simulink model "InitialModel_backup"  (R2020a)
settings: Solver=VariableStepAuto  StartTime=0.0  StopTime=20  RelTol=0.001
values from neighbouring files (symbols this model uses):
  Ax = 0.1    [Simulink1.m]
  Ay = 0.1    [Simulink1.m]
  Az = 0.1    [Simulink1.m]
  g = 9.81    [Simulink1.m]
  Ixx = 0.00365    [Simulink1.m]
  Iyy = 0.00368    [Simulink1.m]
  Izz = 0.00703    [Simulink1.m]
  Jyy = 0.0064    [Simulink1.m]
  k_F = 6.11e-8    (= 6.11e-08)    [Simulink1.m]
  k_M = 1.5e-9    (= 1.5e-09)    [Simulink1.m]
  l = 0.17    [Simulink1.m]
  m = 0.5    [Simulink1.m]
settings Model: Creator=o_belzil  LastModifiedBy=o_belzil
settings SolverCC: MaxConsecutiveZCs=10  MaxConsecutiveMinStep=100  ZeroCrossAlgorithm=Adaptive
settings DebuggingCC: MaskedZcDiagnostic=none  IgnoredZcDiagnostic=none  UniqueDataStoreMsg=error

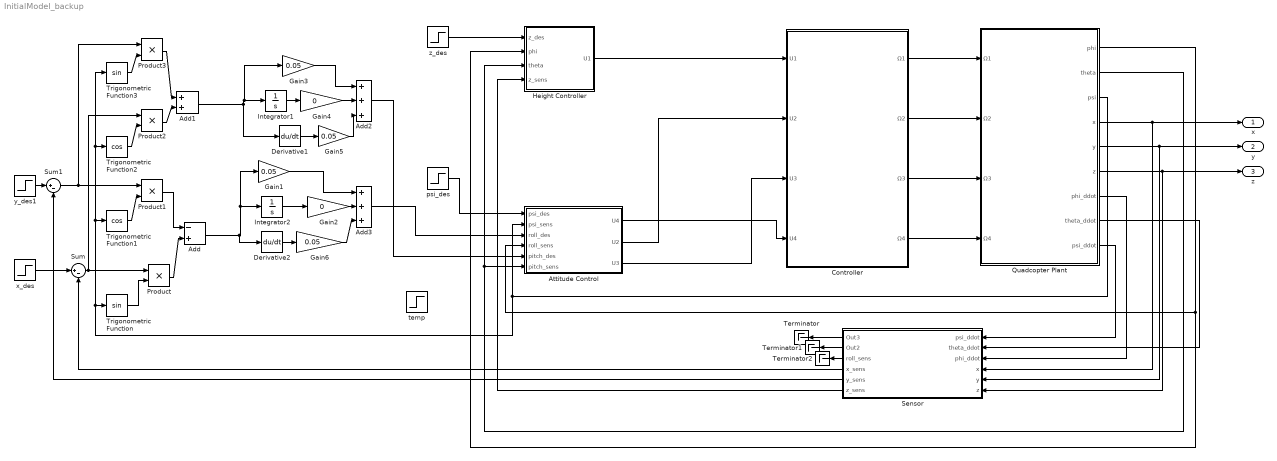
== system InitialModel_backup ==
  Add : Sum  Inputs=-+
  Add1 : Sum
  Add2 : Sum  Inputs=+++
  Add3 : Sum  Inputs=+++
  Attitude Control : Subsystem
  Controller : Subsystem
  Derivative1 : Derivative
  Derivative2 : Derivative
  Gain{1,3,5..6} (4 alike) : Gain  Gain=0.05
  Gain2 : Gain  Gain=0
  Gain4 : Gain  Gain=0
  Height Controller : Subsystem
  Integrator1 : Integrator
  Integrator2 : Integrator
  Product{,1..3} (4 alike) : Product
  Quadcopter Plant : Subsystem
  Sensor : Subsystem
  Sum : Sum  Inputs=|+-
  Sum1 : Sum  Inputs=|+-
  Terminator : Terminator
  Terminator1 : Terminator
  Terminator2 : Terminator
  Trigonometric Function : Trigonometry
  Trigonometric Function1 : Trigonometry  Operator=cos
  Trigonometric Function2 : Trigonometry  Operator=cos
  Trigonometric Function3 : Trigonometry
  psi_des : Step  Time=0  After=1.6  SampleTime=0
  temp : Step  Time=0  After=0.75  SampleTime=0
  x_des : Step  Time=2  After=5  SampleTime=0
  y_des1 : Step  Time=0  After=0  SampleTime=0
  z_des : Step  Time=0  After=10  SampleTime=0
  x : Outport
  y : Outport  Port=2
  z : Outport  Port=3
  wires:
  Quadcopter Plant/4(x) -> x/1, Sensor/4(x)
  Quadcopter Plant/5(y) -> y/1, Sensor/5(y)
  Quadcopter Plant/6(z) -> z/1, Sensor/6(z)
  Quadcopter Plant/7(phi_ddot) -> Sensor/3(phi_ddot)
  Quadcopter Plant/8(theta_ddot) -> Sensor/2(theta_ddot)
  Controller/1(Ω1) -> Quadcopter Plant/1(Ω1)
  Controller/2(Ω2) -> Quadcopter Plant/2(Ω2)
  Controller/3(Ω3) -> Quadcopter Plant/3(Ω3)
  Controller/4(Ω4) -> Quadcopter Plant/4(Ω4)
  Height Controller/1(U1) -> Controller/1(U1)
  z_des/1 -> Height Controller/1(z_des)
  Quadcopter Plant/1(phi) -> Attitude Control/4(roll_sens), Height Controller/2(phi)
  Quadcopter Plant/2(theta) -> Attitude Control/6(pitch_sens), Height Controller/3(theta)
  psi_des/1 -> Attitude Control/1(psi_des)
  Quadcopter Plant/3(psi) -> Attitude Control/2(psi_sens), Trigonometric Function3/1, Trigonometric Function2/1, Trigonometric Function1/1, Trigonometric Function/1
  Attitude Control/1(U4) -> Controller/4(U4)
  Sensor/6(z_sens) -> Height Controller/4(z_sens)
  Attitude Control/2(U2) -> Controller/2(U2)
  Attitude Control/3(U3) -> Controller/3(U3)
  x_des/1 -> Sum/1
  Sensor/4(x_sens) -> Sum/2
  Sum/1 -> Product/1, Product2/1
  Trigonometric Function/1 -> Product/2
  Product/1 -> Add/2
  y_des1/1 -> Sum1/1
  Sensor/5(y_sens) -> Sum1/2
  Sum1/1 -> Product1/1, Product3/1
  Trigonometric Function1/1 -> Product1/2
  Product1/1 -> Add/1
  Trigonometric Function2/1 -> Product2/2
  Trigonometric Function3/1 -> Product3/2
  Product3/1 -> Add1/1
  Product2/1 -> Add1/2
  Integrator1/1 -> Gain4/1
  Gain5/1 -> Add2/3
  Gain4/1 -> Add2/2
  Add1/1 -> Integrator1/1, Gain3/1, Derivative1/1
  Gain3/1 -> Add2/1
  Derivative1/1 -> Gain5/1
  Integrator2/1 -> Gain2/1
  Gain6/1 -> Add3/3
  Gain2/1 -> Add3/2
  Add/1 -> Derivative2/1, Integrator2/1, Gain1/1
  Gain1/1 -> Add3/1
  Derivative2/1 -> Gain6/1
  Sensor/2(Out2) -> Terminator1/1
  Sensor/3(roll_sens) -> Terminator2/1
  Sensor/1(Out3) -> Terminator/1
  Quadcopter Plant/9(psi_ddot) -> Sensor/1(psi_ddot)
  Add3/1 -> Attitude Control/3(roll_des)
  Add2/1 -> Attitude Control/5(pitch_des)

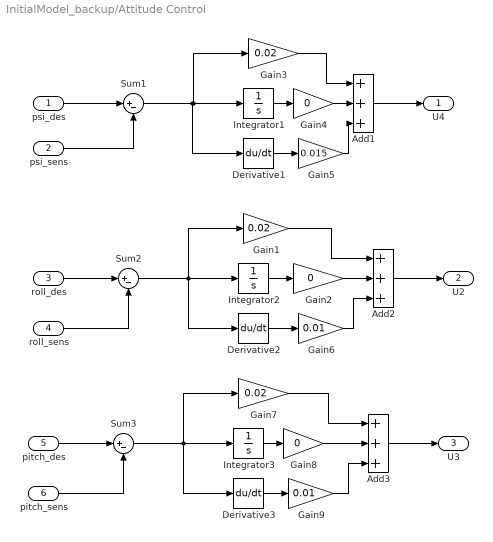
== system InitialModel_backup/Attitude Control ==
  psi_des : Inport
  psi_sens : Inport  Port=2
  roll_des : Inport  Port=3
  roll_sens : Inport  Port=4
  pitch_des : Inport  Port=5
  pitch_sens : Inport  Port=6
  Add1 : Sum  Inputs=+++
  Add2 : Sum  Inputs=+++
  Add3 : Sum  Inputs=+++
  Derivative1 : Derivative
  Derivative2 : Derivative
  Derivative3 : Derivative
  Gain1 : Gain  Gain=0.02
  Gain2 : Gain  Gain=0
  Gain3 : Gain  Gain=0.02
  Gain4 : Gain  Gain=0
  Gain5 : Gain  Gain=0.015
  Gain6 : Gain  Gain=0.01
  Gain7 : Gain  Gain=0.02
  Gain8 : Gain  Gain=0
  Gain9 : Gain  Gain=0.01
  Integrator1 : Integrator
  Integrator2 : Integrator
  Integrator3 : Integrator
  Sum1 : Sum  Inputs=|+-
  Sum2 : Sum  Inputs=|+-
  Sum3 : Sum  Inputs=|+-
  U4 : Outport
  U2 : Outport  Port=2
  U3 : Outport  Port=3
  wires:
  Gain3/1 -> Add1/1
  Gain4/1 -> Add1/2
  Gain5/1 -> Add1/3
  Derivative1/1 -> Gain5/1
  Integrator1/1 -> Gain4/1
  Add1/1 -> U4/1
  psi_des/1 -> Sum1/1
  psi_sens/1 -> Sum1/2
  Sum1/1 -> Derivative1/1, Integrator1/1, Gain3/1
  Integrator2/1 -> Gain2/1
  Gain6/1 -> Add2/3
  Gain2/1 -> Add2/2
  Add2/1 -> U2/1
  Sum2/1 -> Derivative2/1, Integrator2/1, Gain1/1
  roll_des/1 -> Sum2/1
  Gain1/1 -> Add2/1
  Derivative2/1 -> Gain6/1
  roll_sens/1 -> Sum2/2
  pitch_sens/1 -> Sum3/2
  Gain7/1 -> Add3/1
  Add3/1 -> U3/1
  Gain9/1 -> Add3/3
  Sum3/1 -> Derivative3/1, Integrator3/1, Gain7/1
  Integrator3/1 -> Gain8/1
  pitch_des/1 -> Sum3/1
  Gain8/1 -> Add3/2
  Derivative3/1 -> Gain9/1

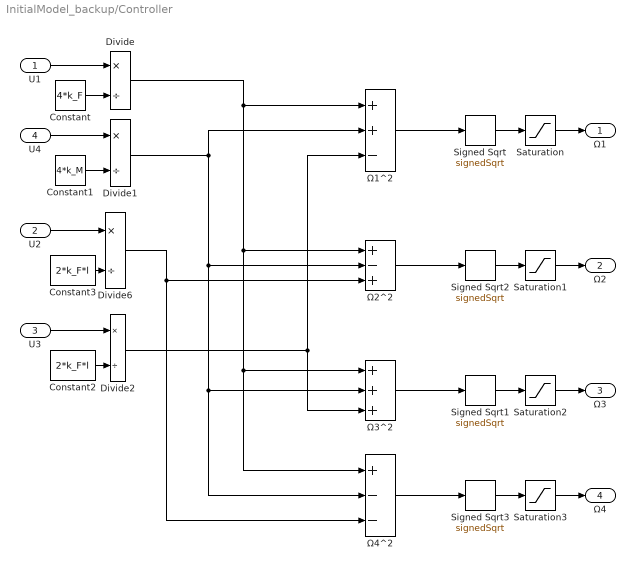
== system InitialModel_backup/Controller ==
  U1 : Inport
  U2 : Inport  Port=2
  U3 : Inport  Port=3
  U4 : Inport  Port=4
  Constant : Constant  Value=4*k_F
  Constant1 : Constant  Value=4*k_M
  Constant2 : Constant  Value=2*k_F*l
  Constant3 : Constant  Value=2*k_F*l
  Divide{,1..2,6} (4 alike) : Product  Inputs=*/
  Saturation{,1..3} (4 alike) : Saturate  UpperLimit=10000  LowerLimit=0
  Signed Sqrt{,1..3} (4 alike) : Sqrt  Operator=signedSqrt  SaturateOnIntegerOverflow=on
  Ω1^2 : Sum  Inputs=++-
  Ω2^2 : Sum  Inputs=+-+
  Ω3^2 : Sum  Inputs=+++
  Ω4^2 : Sum  Inputs=+--
  Ω1 : Outport
  Ω2 : Outport  Port=2
  Ω3 : Outport  Port=3
  Ω4 : Outport  Port=4
  wires:
  Ω1^2/1 -> Signed Sqrt/1
  Ω3^2/1 -> Signed Sqrt1/1
  Ω4^2/1 -> Signed Sqrt3/1
  Ω2^2/1 -> Signed Sqrt2/1
  U1/1 -> Divide/1
  Constant/1 -> Divide/2
  U4/1 -> Divide1/1
  Constant1/1 -> Divide1/2
  Constant2/1 -> Divide2/2
  U3/1 -> Divide2/1
  Constant3/1 -> Divide6/2
  U2/1 -> Divide6/1
  Divide/1 -> Ω4^2/1, Ω3^2/1, Ω2^2/1, Ω1^2/1
  Divide1/1 -> Ω4^2/2, Ω3^2/2, Ω2^2/2, Ω1^2/2
  Divide2/1 -> Ω3^2/3, Ω1^2/3
  Divide6/1 -> Ω4^2/3, Ω2^2/3
  Signed Sqrt3/1 -> Saturation3/1
  Saturation3/1 -> Ω4/1
  Signed Sqrt1/1 -> Saturation2/1
  Saturation2/1 -> Ω3/1
  Signed Sqrt2/1 -> Saturation1/1
  Saturation1/1 -> Ω2/1
  Signed Sqrt/1 -> Saturation/1
  Saturation/1 -> Ω1/1

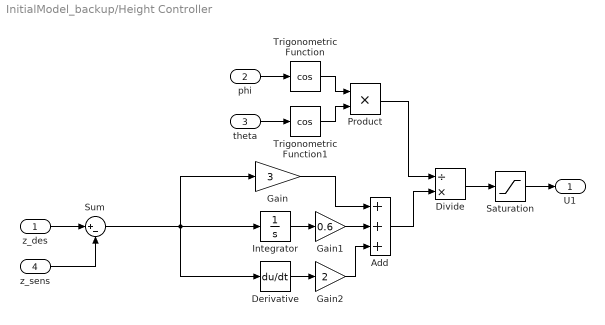
== system InitialModel_backup/Height Controller ==
  z_des : Inport
  phi : Inport  Port=2
  theta : Inport  Port=3
  z_sens : Inport  Port=4
  Add : Sum  Inputs=+++
  Derivative : Derivative
  Divide : Product  Inputs=/*
  Gain : Gain  Gain=3
  Gain1 : Gain  Gain=0.6
  Gain2 : Gain  Gain=2
  Integrator : Integrator
  Product : Product
  Saturation : Saturate  UpperLimit=inf  LowerLimit=0
  Sum : Sum  Inputs=|+-
  Trigonometric Function : Trigonometry  Operator=cos
  Trigonometric Function1 : Trigonometry  Operator=cos
  U1 : Outport
  wires:
  Integrator/1 -> Gain1/1
  Gain1/1 -> Add/2
  Trigonometric Function1/1 -> Product/2
  Derivative/1 -> Gain2/1
  Divide/1 -> Saturation/1
  Trigonometric Function/1 -> Product/1
  Gain/1 -> Add/1
  Product/1 -> Divide/1
  Gain2/1 -> Add/3
  Saturation/1 -> U1/1
  z_des/1 -> Sum/1
  z_sens/1 -> Sum/2
  phi/1 -> Trigonometric Function/1
  theta/1 -> Trigonometric Function1/1
  Sum/1 -> Integrator/1, Derivative/1, Gain/1
  Add/1 -> Divide/2

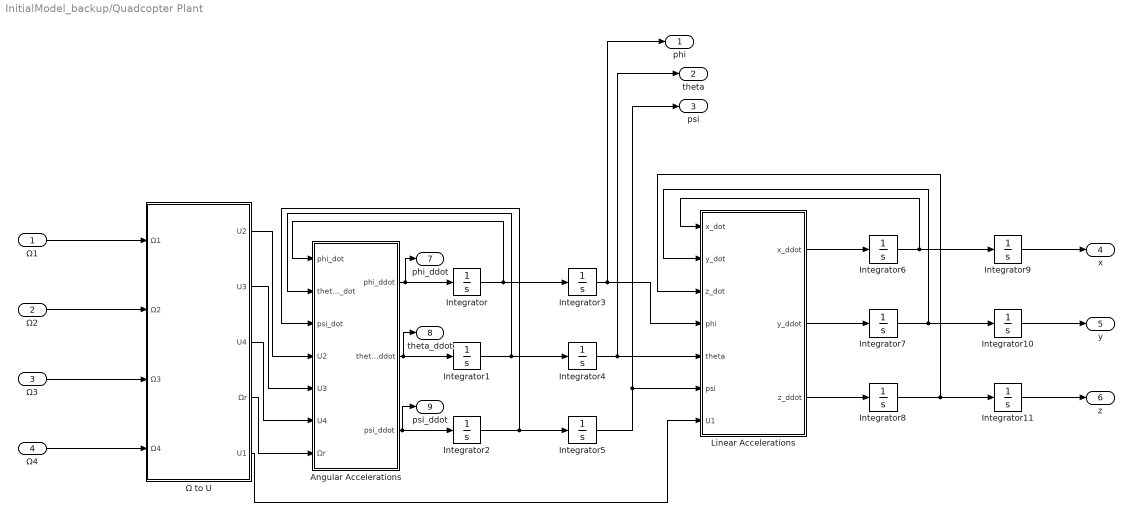
== system InitialModel_backup/Quadcopter Plant ==
  Ω1 : Inport
  Ω2 : Inport  Port=2
  Ω3 : Inport  Port=3
  Ω4 : Inport  Port=4
  Angular Accelerations : Subsystem
  Integrator{,1..2,6..10} (8 alike) : Integrator
  Integrator11 : Integrator  LimitOutput=on  LowerSaturationLimit=0
  Integrator3 : Integrator  WrapState=on
  Integrator4 : Integrator  WrapState=on
  Integrator5 : Integrator  WrapState=on
  Linear Accelerations : Subsystem
  Ω to U : Subsystem
  phi : Outport
  theta : Outport  Port=2
  psi : Outport  Port=3
  x : Outport  Port=4
  y : Outport  Port=5
  z : Outport  Port=6
  phi_ddot : Outport  Port=7
  theta_ddot : Outport  Port=8
  psi_ddot : Outport  Port=9
  wires:
  Ω1/1 -> Ω to U/1(Ω1)
  Ω2/1 -> Ω to U/2(Ω2)
  Ω3/1 -> Ω to U/3(Ω3)
  Ω4/1 -> Ω to U/4(Ω4)
  Ω to U/1(U2) -> Angular Accelerations/4(U2)
  Ω to U/2(U3) -> Angular Accelerations/5(U3)
  Ω to U/3(U4) -> Angular Accelerations/6(U4)
  Ω to U/4(Ωr) -> Angular Accelerations/7(Ωr)
  Angular Accelerations/3(psi_ddot) -> psi_ddot/1, Integrator2/1
  Angular Accelerations/2(theta_ddot) -> Integrator1/1, theta_ddot/1
  Angular Accelerations/1(phi_ddot) -> phi_ddot/1, Integrator/1
  Integrator/1 -> Integrator3/1, Angular Accelerations/1(phi_dot)
  Integrator1/1 -> Integrator4/1, Angular Accelerations/2(theta_dot)
  Integrator2/1 -> Integrator5/1, Angular Accelerations/3(psi_dot)
  Integrator3/1 -> Linear Accelerations/4(phi), phi/1
  Integrator4/1 -> Linear Accelerations/5(theta), theta/1
  Integrator5/1 -> psi/1, Linear Accelerations/6(psi)
  Linear Accelerations/1(x_ddot) -> Integrator6/1
  Linear Accelerations/2(y_ddot) -> Integrator7/1
  Linear Accelerations/3(z_ddot) -> Integrator8/1
  Integrator6/1 -> Integrator9/1, Linear Accelerations/1(x_dot)
  Integrator7/1 -> Integrator10/1, Linear Accelerations/2(y_dot)
  Integrator8/1 -> Integrator11/1, Linear Accelerations/3(z_dot)
  Integrator9/1 -> x/1
  Integrator10/1 -> y/1
  Integrator11/1 -> z/1
  Ω to U/5(U1) -> Linear Accelerations/7(U1)

== system InitialModel_backup/Sensor ==
  psi_ddot : Inport
  theta_ddot : Inport  Port=2
  phi_ddot : Inport  Port=3
  x : Inport  Port=4
  y : Inport  Port=5
  z : Inport  Port=6
  Out3 : Outport
  Out2 : Outport  Port=2
  roll_sens : Outport  Port=3
  x_sens : Outport  Port=4
  y_sens : Outport  Port=5
  z_sens : Outport  Port=6
  wires:
  phi_ddot/1 -> roll_sens/1
  theta_ddot/1 -> Out2/1
  psi_ddot/1 -> Out3/1
  x/1 -> x_sens/1
  z/1 -> z_sens/1
  y/1 -> y_sens/1

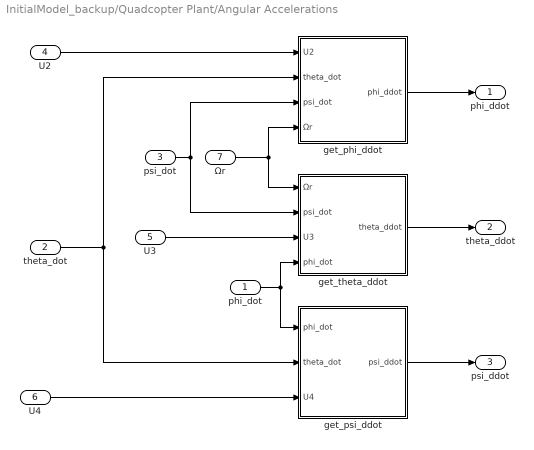
== system InitialModel_backup/Quadcopter Plant/Angular Accelerations ==
  phi_dot : Inport
  theta_dot : Inport  Port=2
  psi_dot : Inport  Port=3
  U2 : Inport  Port=4
  U3 : Inport  Port=5
  U4 : Inport  Port=6
  Ωr : Inport  Port=7
  get_phi_ddot : Subsystem
  get_psi_ddot : Subsystem
  get_theta_ddot : Subsystem
  phi_ddot : Outport
  theta_ddot : Outport  Port=2
  psi_ddot : Outport  Port=3
  wires:
  get_phi_ddot/1(phi_ddot) -> phi_ddot/1
  get_theta_ddot/1(theta_ddot) -> theta_ddot/1
  get_psi_ddot/1(psi_ddot) -> psi_ddot/1
  U2/1 -> get_phi_ddot/1(U2)
  U4/1 -> get_psi_ddot/3(U4)
  Ωr/1 -> get_theta_ddot/1(Ωr), get_phi_ddot/4(Ωr)
  psi_dot/1 -> get_theta_ddot/2(psi_dot), get_phi_ddot/3(psi_dot)
  phi_dot/1 -> get_psi_ddot/1(phi_dot), get_theta_ddot/4(phi_dot)
  theta_dot/1 -> get_psi_ddot/2(theta_dot), get_phi_ddot/2(theta_dot)
  U3/1 -> get_theta_ddot/3(U3)

== system InitialModel_backup/Quadcopter Plant/Linear Accelerations ==
  x_dot : Inport
  y_dot : Inport  Port=2
  z_dot : Inport  Port=3
  phi : Inport  Port=4
  theta : Inport  Port=5
  psi : Inport  Port=6
  U1 : Inport  Port=7
  get_x_ddot : Subsystem
  get_y_ddot : Subsystem
  get_z_ddot : Subsystem
  x_ddot : Outport
  y_ddot : Outport  Port=2
  z_ddot : Outport  Port=3
  wires:
  x_dot/1 -> get_x_ddot/1(x_dot)
  y_dot/1 -> get_y_ddot/1(y_dot)
  z_dot/1 -> get_z_ddot/1(z_dot)
  psi/1 -> get_x_ddot/4(psi), get_y_ddot/4(psi)
  theta/1 -> get_z_ddot/3(theta), get_y_ddot/3(theta), get_x_ddot/3(theta)
  phi/1 -> get_x_ddot/2(phi), get_z_ddot/2(phi), get_y_ddot/2(phi)
  get_z_ddot/1(z_ddot) -> z_ddot/1
  get_y_ddot/1(y_ddot) -> y_ddot/1
  get_x_ddot/1(x_ddot) -> x_ddot/1
  U1/1 -> get_z_ddot/4(U1), get_y_ddot/5(U1), get_x_ddot/5(U1)

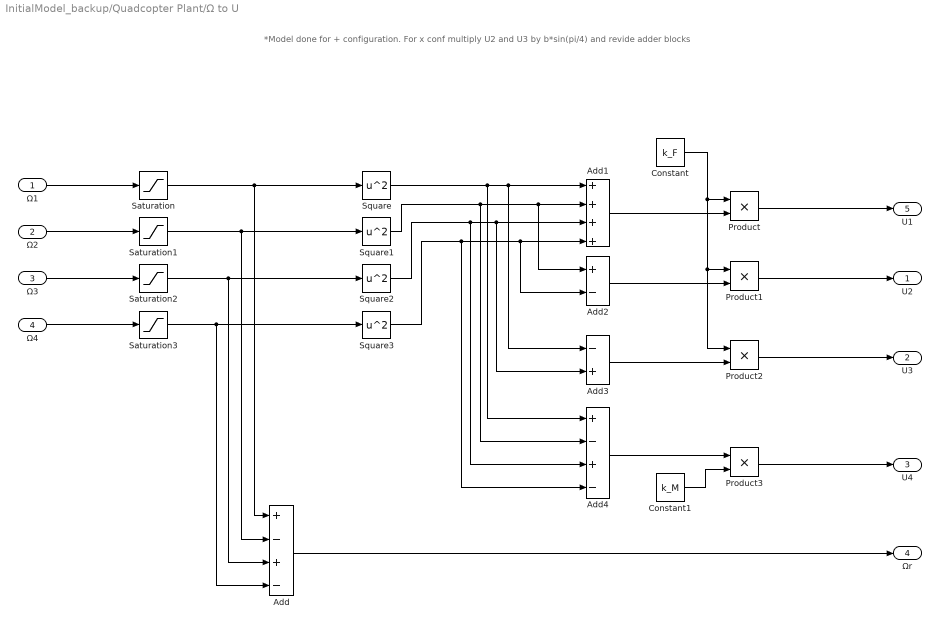
== system InitialModel_backup/Quadcopter Plant/Ω to U ==
  note: *Model done for + configuration. For x conf multiply U2 and U3 by b*sin(pi/4) and revide adder blocks
  Ω1 : Inport
  Ω2 : Inport  Port=2
  Ω3 : Inport  Port=3
  Ω4 : Inport  Port=4
  Add : Sum  Inputs=+-+-
  Add1 : Sum  Inputs=++++
  Add2 : Sum  Inputs=+-
  Add3 : Sum  Inputs=-+
  Add4 : Sum  Inputs=+-+-
  Constant : Constant  Value=k_F
  Constant1 : Constant  Value=k_M
  Product{,1..3} (4 alike) : Product
  Saturation{,1..3} (4 alike) : Saturate  UpperLimit=inf  LowerLimit=0
  Square{,1..3} (4 alike) : Math  Operator=square  SaturateOnIntegerOverflow=on
  U2 : Outport
  U3 : Outport  Port=2
  U4 : Outport  Port=3
  Ωr : Outport  Port=4
  U1 : Outport  Port=5
  wires:
  Ω1/1 -> Saturation/1
  Ω2/1 -> Saturation1/1
  Ω3/1 -> Saturation2/1
  Ω4/1 -> Saturation3/1
  Add/1 -> Ωr/1
  Square/1 -> Add3/1, Add1/1, Add4/1
  Square1/1 -> Add2/1, Add1/2, Add4/2
  Square2/1 -> Add3/2, Add1/3, Add4/3
  Square3/1 -> Add4/4, Add2/2, Add1/4
  Add1/1 -> Product/2
  Add2/1 -> Product1/2
  Add3/1 -> Product2/2
  Add4/1 -> Product3/1
  Constant1/1 -> Product3/2
  Constant/1 -> Product/1, Product2/1, Product1/1
  Product/1 -> U1/1
  Product1/1 -> U2/1
  Product2/1 -> U3/1
  Product3/1 -> U4/1
  Saturation/1 -> Square/1, Add/1
  Saturation1/1 -> Square1/1, Add/2
  Saturation2/1 -> Square2/1, Add/3
  Saturation3/1 -> Square3/1, Add/4

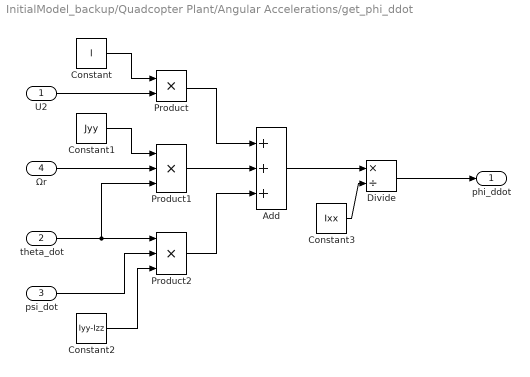
== system InitialModel_backup/Quadcopter Plant/Angular Accelerations/get_phi_ddot ==
  U2 : Inport
  theta_dot : Inport  Port=2
  psi_dot : Inport  Port=3
  Ωr : Inport  Port=4
  Add : Sum  Inputs=+++
  Constant : Constant  Value=l
  Constant1 : Constant  Value=Jyy
  Constant2 : Constant  Value=Iyy-Izz
  Constant3 : Constant  Value=Ixx
  Divide : Product  Inputs=*/
  Product : Product
  Product1 : Product  Inputs=3
  Product2 : Product  Inputs=3
  phi_ddot : Outport
  wires:
  U2/1 -> Product/2
  Constant/1 -> Product/1
  Ωr/1 -> Product1/2
  Constant1/1 -> Product1/1
  theta_dot/1 -> Product2/1, Product1/3
  psi_dot/1 -> Product2/2
  Constant2/1 -> Product2/3
  Product/1 -> Add/1
  Product1/1 -> Add/2
  Product2/1 -> Add/3
  Add/1 -> Divide/1
  Constant3/1 -> Divide/2
  Divide/1 -> phi_ddot/1

== system InitialModel_backup/Quadcopter Plant/Angular Accelerations/get_psi_ddot ==
  phi_dot : Inport
  theta_dot : Inport  Port=2
  U4 : Inport  Port=3
  Add : Sum
  Constant : Constant  Value=Ixx-Iyy
  Constant1 : Constant  Value=Izz
  Divide : Product  Inputs=*/
  Product : Product  Inputs=3
  psi_ddot : Outport
  wires:
  Constant1/1 -> Divide/2
  Add/1 -> Divide/1
  U4/1 -> Add/1
  phi_dot/1 -> Product/1
  theta_dot/1 -> Product/2
  Constant/1 -> Product/3
  Product/1 -> Add/2
  Divide/1 -> psi_ddot/1

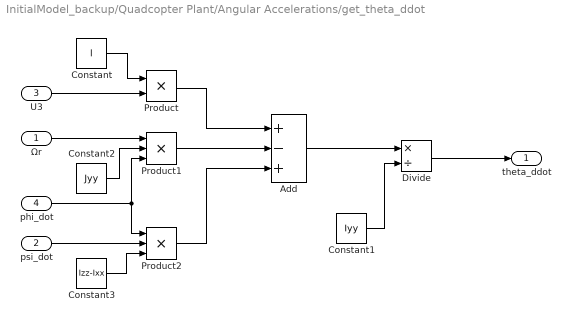
== system InitialModel_backup/Quadcopter Plant/Angular Accelerations/get_theta_ddot ==
  Ωr : Inport
  psi_dot : Inport  Port=2
  U3 : Inport  Port=3
  phi_dot : Inport  Port=4
  Add : Sum  Inputs=+-+
  Constant : Constant  Value=l
  Constant1 : Constant  Value=Iyy
  Constant2 : Constant  Value=Jyy
  Constant3 : Constant  Value=Izz-Ixx
  Divide : Product  Inputs=*/
  Product : Product
  Product1 : Product  Inputs=3
  Product2 : Product  Inputs=3
  theta_ddot : Outport
  wires:
  Constant/1 -> Product/1
  U3/1 -> Product/2
  Ωr/1 -> Product1/1
  phi_dot/1 -> Product2/1, Product1/3
  Constant2/1 -> Product1/2
  Constant3/1 -> Product2/3
  psi_dot/1 -> Product2/2
  Product/1 -> Add/1
  Product1/1 -> Add/2
  Product2/1 -> Add/3
  Add/1 -> Divide/1
  Constant1/1 -> Divide/2
  Divide/1 -> theta_ddot/1

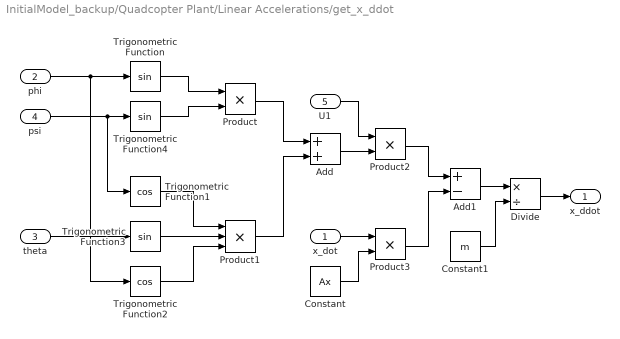
== system InitialModel_backup/Quadcopter Plant/Linear Accelerations/get_x_ddot ==
  x_dot : Inport
  phi : Inport  Port=2
  theta : Inport  Port=3
  psi : Inport  Port=4
  U1 : Inport  Port=5
  Add : Sum
  Add1 : Sum  Inputs=+-
  Constant : Constant  Value=Ax
  Constant1 : Constant  Value=m
  Divide : Product  Inputs=*/
  Product : Product
  Product1 : Product  Inputs=3
  Product2 : Product
  Product3 : Product
  Trigonometric Function : Trigonometry
  Trigonometric Function1 : Trigonometry  Operator=cos
  Trigonometric Function2 : Trigonometry  Operator=cos
  Trigonometric Function3 : Trigonometry
  Trigonometric Function4 : Trigonometry
  x_ddot : Outport
  wires:
  phi/1 -> Trigonometric Function2/1, Trigonometric Function/1
  psi/1 -> Trigonometric Function1/1, Trigonometric Function4/1
  theta/1 -> Trigonometric Function3/1
  Trigonometric Function/1 -> Product/1
  Trigonometric Function4/1 -> Product/2
  Trigonometric Function3/1 -> Product1/2
  Trigonometric Function1/1 -> Product1/1
  Trigonometric Function2/1 -> Product1/3
  Product/1 -> Add/1
  Product1/1 -> Add/2
  Add/1 -> Product2/2
  U1/1 -> Product2/1
  x_dot/1 -> Product3/1
  Constant/1 -> Product3/2
  Product2/1 -> Add1/1
  Product3/1 -> Add1/2
  Add1/1 -> Divide/1
  Constant1/1 -> Divide/2
  Divide/1 -> x_ddot/1

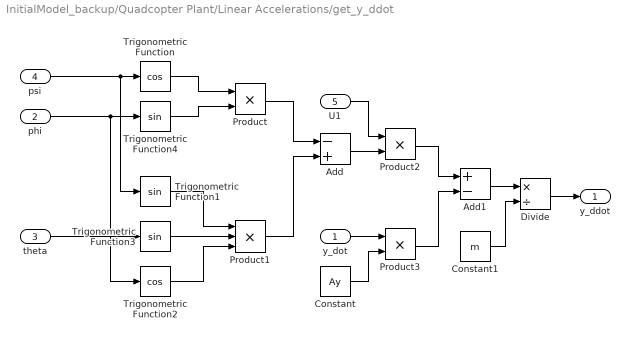
== system InitialModel_backup/Quadcopter Plant/Linear Accelerations/get_y_ddot ==
  y_dot : Inport
  phi : Inport  Port=2
  theta : Inport  Port=3
  psi : Inport  Port=4
  U1 : Inport  Port=5
  Add : Sum  Inputs=-+
  Add1 : Sum  Inputs=+-
  Constant : Constant  Value=Ay
  Constant1 : Constant  Value=m
  Divide : Product  Inputs=*/
  Product : Product
  Product1 : Product  Inputs=3
  Product2 : Product
  Product3 : Product
  Trigonometric Function : Trigonometry  Operator=cos
  Trigonometric Function1 : Trigonometry
  Trigonometric Function2 : Trigonometry  Operator=cos
  Trigonometric Function3 : Trigonometry
  Trigonometric Function4 : Trigonometry
  y_ddot : Outport
  wires:
  Trigonometric Function4/1 -> Product/2
  Trigonometric Function3/1 -> Product1/2
  Trigonometric Function1/1 -> Product1/1
  Add1/1 -> Divide/1
  Product1/1 -> Add/2
  Divide/1 -> y_ddot/1
  y_dot/1 -> Product3/1
  Trigonometric Function/1 -> Product/1
  Product/1 -> Add/1
  Constant/1 -> Product3/2
  Constant1/1 -> Divide/2
  Product2/1 -> Add1/1
  U1/1 -> Product2/1
  Product3/1 -> Add1/2
  Trigonometric Function2/1 -> Product1/3
  Add/1 -> Product2/2
  phi/1 -> Trigonometric Function2/1, Trigonometric Function4/1
  psi/1 -> Trigonometric Function1/1, Trigonometric Function/1
  theta/1 -> Trigonometric Function3/1

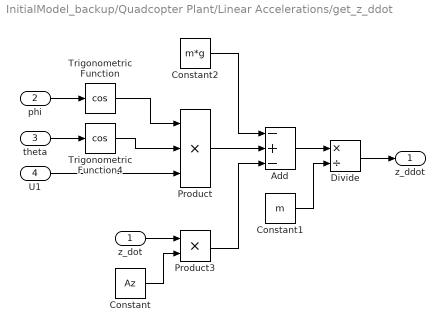
== system InitialModel_backup/Quadcopter Plant/Linear Accelerations/get_z_ddot ==
  z_dot : Inport
  phi : Inport  Port=2
  theta : Inport  Port=3
  U1 : Inport  Port=4
  Add : Sum  Inputs=-+-
  Constant : Constant  Value=Az
  Constant1 : Constant  Value=m
  Constant2 : Constant  Value=m*g
  Divide : Product  Inputs=*/
  Product : Product  Inputs=3
  Product3 : Product
  Trigonometric Function : Trigonometry  Operator=cos
  Trigonometric Function4 : Trigonometry  Operator=cos
  z_ddot : Outport
  wires:
  Trigonometric Function4/1 -> Product/2
  Add/1 -> Divide/1
  Divide/1 -> z_ddot/1
  z_dot/1 -> Product3/1
  Trigonometric Function/1 -> Product/1
  Constant/1 -> Product3/2
  Constant1/1 -> Divide/2
  phi/1 -> Trigonometric Function/1
  theta/1 -> Trigonometric Function4/1
  U1/1 -> Product/3
  Product/1 -> Add/2
  Constant2/1 -> Add/1
  Product3/1 -> Add/3
